simulink model "Validation_Tricopter_Model"  (R2015a)
settings: Solver=ode3  SolverMode=SingleTasking  StartTime=0.0  StopTime=20  FixedStep=T_sim  RelTol=1e-3
PreLoadFcn:
  | LoadLibraries
values from neighbouring files (symbols this model uses):
  a = 10.26    [SetupComplete.m]
  A_x = 0.015    [SetupComplete.m]
  A_y = A_x    (= 0.015)    [SetupComplete.m]
  A_z = 0.16    [SetupComplete.m]
  C_d0 = 0.001193    [SetupComplete.m]
  C_x = 1.2    [SetupComplete.m]
  C_y = C_x    (= 1.2)    [SetupComplete.m]
  C_z = 2.2    [SetupComplete.m]
  CG_0 = [0,0,0.02]'    [SetupComplete.m]
  g = 9.81    [SetupComplete.m]
  h = 0.08    [SetupComplete.m]
  h_FA = 0.02    [SetupComplete.m]
  h_M = 0.064    [SetupComplete.m]
  I_BAC_0 = [ Ix,0,Ixz;0,Iy,0;Ixz,0,Iz]    [SetupComplete.m]
  I_prop = 1/4*M_eq*R^2*diag([1,1,2])    [SetupComplete.m]
  I_tube = [1/2*M_tube*R_tube_eq^2,0,  0  ;           0 ,1/3*M_tube*l_arm^2,0;             0  ,0,1/3*M_tube*l_arm^2]    [SetupComplete.m]
  Initial_Omegas = [1;1;1]*Omega_hover    [Run3Copter.m]
  J_FA = I_prop(1,1) + m_prop*h^2  + m_FA*h_FA^2 + m_M*h_M^2    [SetupComplete.m]
  J_T = J_m+1/2*M_eq*R^2    (= 2.000642e-05)    [SetupComplete.m]
  Ki = lqi(LM_4DOF_aug, Q,R)    [robust_controller.m]
  l = 0.3450    (= 0.345)    [NDI_components.m]    (also in SetupComplete.m; robust_controller.m)
  l_arm = 0.264    [SetupComplete.m]
  m = 3.51    [SetupComplete.m]
  m_0 = 2.61    [SetupComplete.m]
  m_FA = 0.02    [SetupComplete.m]
  m_M = 0.300    (= 0.3)    [SetupComplete.m]
  m_prop = 0.02    [SetupComplete.m]
  R = 0.1778    [SetupComplete.m]    (also in robust_controller.m = eye(4))
  rho = 1.15    [SetupComplete.m]
  sigma = b*c/(pi*R)    (= 0.107416159567)    [SetupComplete.m]
  T_sim = 0.01    [Run3Copter.m]
  theta_0 = 0.38397    [SetupComplete.m]
  theta_1 = -0.2967    [SetupComplete.m]
  trim_simplemodel = [0.589627915568 -2.20656039197 0 0.588313336084 0 0 0.588313330414 0 0]    [trimvalues.mat]
  V_4DOF_last = [0.0122475086001 0.00870447045314 -0.0292257707267 -0.0198753669721 -0.00290766514824 -0.0269511839788 0.0344308792695 -0.0305235710433 -0.0274078219028 -0.0329291952852 -0.0272335702183 -0.00643013158961 ... (1500 elements, 50x30)]    [NN_c_weights.mat]
  v_i0 = sqrt( 1/3*m*g/(2*rho*pi*R^2)  )    [SetupComplete.m]
  W_4DOF_last = [0.0132359246225 -0.0402459595001 -0.0221501781133 0.0046881519205 0.0457506835434 0.0464888535199 -0.0342386918322 0.0470592781761 0.0457166948243 -0.00146243512772 0.0300280468889 -0.0358113661373 ... (204 elements, 4x51)]    [NN_c_weights.mat]
undefined symbols (not defined in the file or in its folder): DOWN_0, EAST_0, Motor, NORTH_0, P_0, Prop, Q_0, R_0, sigmatest, U_0, V_0, v_i_adim, Vx_adim, Vz_adim, W_0
undefined symbols (not defined in the file): Initial_Torques, Rotation_sign, Tau_motors
libraries: simulink x66, XXCopter x32, vrlib x26, simulink_extras x6, Adaptive_FaultTolerantControl x6, qcatlib x4, dspinverses x4, lib_controller x4, aerolib6dofsys x3, aerolibtransform2 x3, aerolib6dof2 x1
(part 7 of 11)

== system Validation_Tricopter_Model/Controller/NDI+CA Controller/4DOF NDI+CA Controller - No massic update/1st order reference model6 ==
  y_ref : Inport
  y_meas : Inport  Port=2
  Bandwidth gain : Gain  Gain=Kb
  Bandwidth gain 1 : Gain  Gain=Kb
  Command FF gain : Gain  Gain=fc
  Command_dot FF gain : Gain  Gain=Kf
  Integral gain : Gain  Gain=fi
  Integrator : Integrator
  Integrator1 : Integrator
  Kref gain : Gain  Gain=Kref
  Sum15 : Sum  Inputs=|+-
  Sum16 : Sum  Inputs=++-
  Sum17 : Sum  Inputs=++|
  Sum5 : Sum  Inputs=|+-
  y_des_dot : Outport
  wires:
  Integral gain/1 -> Integrator1/1
  Bandwidth gain 1/1 -> Integral gain/1
  y_ref/1 -> Sum5/1
  Command_dot FF gain/1 -> Sum17/1
  Command FF gain/1 -> Sum16/1
  Integrator/1 -> Command FF gain/1, Sum15/1, Sum5/2  "y_c"
  y_meas/1 -> Sum16/3, Sum15/2
  Sum16/1 -> Bandwidth gain/1
  Kref gain/1 -> Integrator/1, Command_dot FF gain/1  "y_dot_c"
  Integrator1/1 -> Sum16/2
  Sum17/1 -> y_des_dot/1
  Bandwidth gain/1 -> Sum17/2
  Sum15/1 -> Bandwidth gain 1/1
  Sum5/1 -> Kref gain/1

== system Validation_Tricopter_Model/Controller/NDI+CA Controller/4DOF NDI+CA Controller - No massic update/1st order reference model7 ==
  y_ref : Inport
  y_meas : Inport  Port=2
  Bandwidth gain : Gain  Gain=Kb
  Bandwidth gain 1 : Gain  Gain=Kb
  Command FF gain : Gain  Gain=fc
  Command_dot FF gain : Gain  Gain=Kf
  Integral gain : Gain  Gain=fi
  Integrator : Integrator
  Integrator1 : Integrator
  Kref gain : Gain  Gain=Kref
  Sum15 : Sum  Inputs=|+-
  Sum16 : Sum  Inputs=++-
  Sum17 : Sum  Inputs=++|
  Sum5 : Sum  Inputs=|+-
  y_des_dot : Outport
  wires:
  Sum5/1 -> Kref gain/1
  Sum15/1 -> Bandwidth gain 1/1
  Bandwidth gain/1 -> Sum17/2
  Sum17/1 -> y_des_dot/1
  Integrator1/1 -> Sum16/2
  Kref gain/1 -> Command_dot FF gain/1, Integrator/1  "y_dot_c"
  Sum16/1 -> Bandwidth gain/1
  y_meas/1 -> Sum15/2, Sum16/3
  Integrator/1 -> Sum5/2, Sum15/1, Command FF gain/1  "y_c"
  Command FF gain/1 -> Sum16/1
  Command_dot FF gain/1 -> Sum17/1
  y_ref/1 -> Sum5/1
  Bandwidth gain 1/1 -> Integral gain/1
  Integral gain/1 -> Integrator1/1

== system Validation_Tricopter_Model/Controller/NDI+CA Controller/4DOF NDI+CA Controller - No massic update/Control Allocation 4DOF ==
  Pseudocontrol input : Inport
  Effectiveness control matrix : Inport  Port=2
  Control Allocation 4DOF : Subsystem  VariantControl=(default)
  Pseudoinverse : Subsystem  VariantControl=Variant1
  Control output : Outport

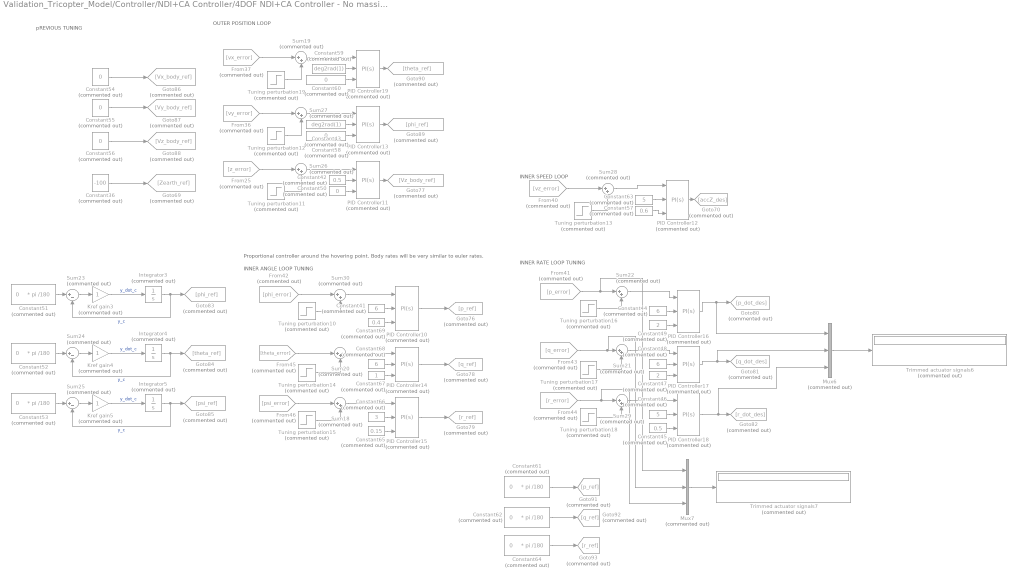
== system Validation_Tricopter_Model/Controller/NDI+CA Controller/4DOF NDI+CA Controller - No massic update/Ideal 4DOF controller ==
  note: OUTER POSITION LOOP
  note: Proportional controller around the hovering point. Body rates will be very similar to euler rates.
  note: INNER RATE LOOP TUNING
  note: INNER ANGLE LOOP TUNING
  note: INNER SPEED LOOP
  note: pREVIOUS TUNING
  Constant36 : Constant  Commented=on  Value=-100
  Constant{41,44,48,68} (4 alike) : Constant  Commented=on  Value=6
  Constant42 : Constant  Commented=on  Value=0.5
  Constant43 : Constant  Commented=on  Value=deg2rad(1)
  Constant45 : Constant  Commented=on  Value=0.5
  Constant46 : Constant  Commented=on  Value=5
  Constant47 : Constant  Commented=on  Value=2
  Constant49 : Constant  Commented=on  Value=2
  Constant{50,54..56,58,60} (6 alike) : Constant  Commented=on  Value=0
  Constant{51..53,61..62,64} (6 alike) : Constant  Commented=on  Value="0     * pi /180"
  Constant57 : Constant  Commented=on  Value=0.6
  Constant59 : Constant  Commented=on  Value=deg2rad(1)
  Constant63 : Constant  Commented=on  Value=5
  Constant65 : Constant  Commented=on  Value=0.15
  Constant66 : Constant  Commented=on  Value=3
  Constant67 : Constant  Commented=on
  Constant69 : Constant  Commented=on  Value=0.4
  From25 : From  Commented=on  GotoTag=z_error
  From36 : From  Commented=on  GotoTag=vy_error
  From37 : From  Commented=on  GotoTag=vx_error
  From40 : From  Commented=on  GotoTag=vz_error
  From41 : From  Commented=on  GotoTag=p_error
  From42 : From  Commented=on  GotoTag=phi_error
  From43 : From  Commented=on  GotoTag=q_error
  From44 : From  Commented=on  GotoTag=r_error
  From45 : From  Commented=on  GotoTag=theta_error
  From46 : From  Commented=on  GotoTag=psi_error
  Goto69 : Goto  Commented=on  GotoTag=Zearth_ref
  Goto70 : Goto  Commented=on  GotoTag=accZ_des
  Goto76 : Goto  Commented=on  GotoTag=p_ref
  Goto77 : Goto  Commented=on  GotoTag=Vz_body_ref
  Goto78 : Goto  Commented=on  GotoTag=q_ref
  Goto79 : Goto  Commented=on  GotoTag=r_ref
  Goto80 : Goto  Commented=on  GotoTag=p_dot_des
  Goto81 : Goto  Commented=on  GotoTag=q_dot_des
  Goto82 : Goto  Commented=on  GotoTag=r_dot_des
  Goto83 : Goto  Commented=on  GotoTag=phi_ref
  Goto84 : Goto  Commented=on  GotoTag=theta_ref
  Goto85 : Goto  Commented=on  GotoTag=psi_ref
  Goto86 : Goto  Commented=on  GotoTag=Vx_body_ref
  Goto87 : Goto  Commented=on  GotoTag=Vy_body_ref
  Goto88 : Goto  Commented=on  GotoTag=Vz_body_ref
  Goto89 : Goto  Commented=on  GotoTag=phi_ref
  Goto90 : Goto  Commented=on  GotoTag=theta_ref
  Goto91 : Goto  Commented=on  GotoTag=p_ref
  Goto92 : Goto  Commented=on  GotoTag=q_ref
  Goto93 : Goto  Commented=on  GotoTag=r_ref
  Integrator3 : Integrator  Commented=on
  Integrator4 : Integrator  Commented=on
  Integrator5 : Integrator  Commented=on
  Kref gain3 : Gain  Commented=on
  Kref gain4 : Gain  Commented=on
  Kref gain5 : Gain  Commented=on
  Mux6 : Mux  Commented=on  Inputs=3
  Mux7 : Mux  Commented=on  Inputs=3
  PID Controller{10..15,18..19} (8 alike) : simulink/Continuous/PID Controller  Commented=on  Controller=PI  TimeDomain=Continuous-time  SampleTime=-1  IntegratorMethod=Forward Euler  FilterMethod=Forward Euler  Form=Parallel  UseFilter=on  ControllerParametersSource=external  P=1  I=1  D=0  N=100  InitialConditionSource=internal  InitialConditionForIntegrator=0  InitialConditionForFilter=0  ExternalReset=none  LimitOutput=off  UpperSaturationLimit=inf  LowerSaturationLimit=-inf  LinearizeAsGain=on  AntiWindupMode=none  Kb=1  TrackingMode=off  Kt=1  PParamMin=[]  PParamMax=[]  IParamMin=[]  IParamMax=[]  DParamMin=[]  DParamMax=[]  NParamMin=[]  NParamMax=[]  KbParamMin=[]  KbParamMax=[]  KtParamMin=[]  KtParamMax=[]  POutMin=[]  POutMax=[]  IOutMin=[]  IOutMax=[]  DOutMin=[]  DOutMax=[]  NOutMin=[]  NOutMax=[]  KbOutMin=[]  KbOutMax=[]  KtOutMin=[]  KtOutMax=[]  IntegratorOutMin=[]  IntegratorOutMax=[]  FilterOutMin=[]  FilterOutMax=[]  SumOutMin=[]  SumOutMax=[]  SumI1OutMin=[]  SumI1OutMax=[]  SumI2OutMin=[]  SumI2OutMax=[]  SumI3OutMin=[]  SumI3OutMax=[]  SumDOutMin=[]  SumDOutMax=[]  SaturationOutMin=[]  SaturationOutMax=[]  IntegratorContinuousStateAttributes=''  IntegratorStateMustResolveToSignalObject=off  IntegratorRTWStateStorageClass=Auto  FilterContinuousStateAttributes=''  FilterStateMustResolveToSignalObject=off  FilterRTWStateStorageClass=Auto  DifferentiatorICPrevScaledInput=0  DifferentiatorOutMin=[]  DifferentiatorOutMax=[]
  PID Controller16 : simulink/Continuous/PID Controller  Commented=on  Controller=PI  TimeDomain=Continuous-time  SampleTime=-1  IntegratorMethod=Forward Euler  FilterMethod=Forward Euler  Form=Parallel  UseFilter=on  ControllerParametersSource=external  P=121.80671459326  I=327.532586687046  D=0  N=100  InitialConditionSource=internal  InitialConditionForIntegrator=0  InitialConditionForFilter=0  ExternalReset=none  LimitOutput=off  UpperSaturationLimit=inf  LowerSaturationLimit=-inf  LinearizeAsGain=on  AntiWindupMode=none  Kb=1  TrackingMode=off  Kt=1  PParamMin=[]  PParamMax=[]  IParamMin=[]  IParamMax=[]  DParamMin=[]  DParamMax=[]  NParamMin=[]  NParamMax=[]  KbParamMin=[]  KbParamMax=[]  KtParamMin=[]  KtParamMax=[]  POutMin=[]  POutMax=[]  IOutMin=[]  IOutMax=[]  DOutMin=[]  DOutMax=[]  NOutMin=[]  NOutMax=[]  KbOutMin=[]  KbOutMax=[]  KtOutMin=[]  KtOutMax=[]  IntegratorOutMin=[]  IntegratorOutMax=[]  FilterOutMin=[]  FilterOutMax=[]  SumOutMin=[]  SumOutMax=[]  SumI1OutMin=[]  SumI1OutMax=[]  SumI2OutMin=[]  SumI2OutMax=[]  SumI3OutMin=[]  SumI3OutMax=[]  SumDOutMin=[]  SumDOutMax=[]  SaturationOutMin=[]  SaturationOutMax=[]  IntegratorContinuousStateAttributes=''  IntegratorStateMustResolveToSignalObject=off  IntegratorRTWStateStorageClass=Auto  FilterContinuousStateAttributes=''  FilterStateMustResolveToSignalObject=off  FilterRTWStateStorageClass=Auto  DifferentiatorICPrevScaledInput=0  DifferentiatorOutMin=[]  DifferentiatorOutMax=[]
  PID Controller17 : simulink/Continuous/PID Controller  Commented=on  Controller=PI  TimeDomain=Continuous-time  SampleTime=-1  IntegratorMethod=Forward Euler  FilterMethod=Forward Euler  Form=Parallel  UseFilter=on  ControllerParametersSource=external  P=244.169484479421  I=1759.80724182952  D=0  N=100  InitialConditionSource=internal  InitialConditionForIntegrator=0  InitialConditionForFilter=0  ExternalReset=none  LimitOutput=off  UpperSaturationLimit=inf  LowerSaturationLimit=-inf  LinearizeAsGain=on  AntiWindupMode=none  Kb=1  TrackingMode=off  Kt=1  PParamMin=[]  PParamMax=[]  IParamMin=[]  IParamMax=[]  DParamMin=[]  DParamMax=[]  NParamMin=[]  NParamMax=[]  KbParamMin=[]  KbParamMax=[]  KtParamMin=[]  KtParamMax=[]  POutMin=[]  POutMax=[]  IOutMin=[]  IOutMax=[]  DOutMin=[]  DOutMax=[]  NOutMin=[]  NOutMax=[]  KbOutMin=[]  KbOutMax=[]  KtOutMin=[]  KtOutMax=[]  IntegratorOutMin=[]  IntegratorOutMax=[]  FilterOutMin=[]  FilterOutMax=[]  SumOutMin=[]  SumOutMax=[]  SumI1OutMin=[]  SumI1OutMax=[]  SumI2OutMin=[]  SumI2OutMax=[]  SumI3OutMin=[]  SumI3OutMax=[]  SumDOutMin=[]  SumDOutMax=[]  SaturationOutMin=[]  SaturationOutMax=[]  IntegratorContinuousStateAttributes=''  IntegratorStateMustResolveToSignalObject=off  IntegratorRTWStateStorageClass=Auto  FilterContinuousStateAttributes=''  FilterStateMustResolveToSignalObject=off  FilterRTWStateStorageClass=Auto  DifferentiatorICPrevScaledInput=0  DifferentiatorOutMin=[]  DifferentiatorOutMax=[]
  Sum{18..22,26..30} (10 alike) : Sum  Commented=on  Inputs=|++
  Sum23 : Sum  Commented=on  Inputs=|+-
  Sum24 : Sum  Commented=on  Inputs=|+-
  Sum25 : Sum  Commented=on  Inputs=|+-
  Trimmed actuator signals6 : Display  Commented=on
  Trimmed actuator signals7 : Display  Commented=on
  Tuning perturbation{10,15..16,18} (4 alike) : Step  Commented=on  Time=20  After=3*pi/180  SampleTime=0
  Tuning perturbation{11..13,19} (4 alike) : Step  Commented=on  Time=20  SampleTime=0
  Tuning perturbation14 : Step  Commented=on  Time=20  After=-3*pi/180  SampleTime=0
  Tuning perturbation17 : Step  Commented=on  Time=20  After=-3*pi/180  SampleTime=0
  wires:
  From42/1 -> Sum30/1
  Constant56/1 -> Goto88/1
  Constant55/1 -> Goto87/1
  Constant54/1 -> Goto86/1
  PID Controller12/1 -> Goto70/1
  Mux6/1 -> Trimmed actuator signals6/1
  Tuning perturbation17/1 -> Sum21/2
  Constant59/1 -> PID Controller19/2
  PID Controller13/1 -> Goto89/1
  Tuning perturbation12/1 -> Sum27/2
  From36/1 -> Sum27/1
  Sum27/1 -> PID Controller13/1
  Constant58/1 -> PID Controller13/3
  PID Controller16/1 -> Goto80/1, Mux6/1
  Tuning perturbation14/1 -> Sum20/2
  Tuning perturbation10/1 -> Sum30/2
  Tuning perturbation15/1 -> Sum18/2
  Sum20/1 -> PID Controller14/1
  Constant66/1 -> PID Controller15/2
  PID Controller15/1 -> Goto79/1
  PID Controller14/1 -> Goto78/1
  PID Controller10/1 -> Goto76/1
  Tuning perturbation13/1 -> Sum28/2
  From40/1 -> Sum28/1
  Constant52/1 -> Sum24/1
  Constant61/1 -> Goto91/1
  Constant45/1 -> PID Controller18/3
  Constant49/1 -> PID Controller16/3
  Sum25/1 -> Kref gain5/1
  Kref gain5/1 -> Integrator5/1  "y_dot_c"
  From43/1 -> Sum21/1, Mux7/2
  From41/1 -> Sum22/1, Mux7/1
  From46/1 -> Sum18/1
  From45/1 -> Sum20/1
  Sum28/1 -> PID Controller12/1
  Constant57/1 -> PID Controller12/3
  Constant63/1 -> PID Controller12/2
  Constant64/1 -> Goto93/1
  Constant62/1 -> Goto92/1
  Constant42/1 -> PID Controller11/2
  Constant36/1 -> Goto69/1
  Constant44/1 -> PID Controller16/2
  Mux7/1 -> Trimmed actuator signals7/1
  From44/1 -> Sum29/1, Mux7/3
  Constant48/1 -> PID Controller17/2
  Constant46/1 -> PID Controller18/2
  PID Controller18/1 -> Goto82/1, Mux6/3
  PID Controller17/1 -> Goto81/1, Mux6/2
  Integrator3/1 -> Goto83/1, Sum23/2  "y_c"
  Constant51/1 -> Sum23/1
  PID Controller19/1 -> Goto90/1
  Tuning perturbation19/1 -> Sum19/2
  From37/1 -> Sum19/1
  Sum19/1 -> PID Controller19/1
  Constant60/1 -> PID Controller19/3
  Constant43/1 -> PID Controller13/2
  PID Controller11/1 -> Goto77/1
  Tuning perturbation11/1 -> Sum26/2
  From25/1 -> Sum26/1
  Sum26/1 -> PID Controller11/1
  Constant50/1 -> PID Controller11/3
  Integrator5/1 -> Goto85/1, Sum25/2  "y_c"
  Constant53/1 -> Sum25/1
  Sum24/1 -> Kref gain4/1
  Kref gain4/1 -> Integrator4/1  "y_dot_c"
  Sum23/1 -> Kref gain3/1
  Kref gain3/1 -> Integrator3/1  "y_dot_c"
  Tuning perturbation16/1 -> Sum22/2
  Tuning perturbation18/1 -> Sum29/2
  Sum21/1 -> PID Controller17/1
  Sum29/1 -> PID Controller18/1
  Sum22/1 -> PID Controller16/1
  Constant47/1 -> PID Controller17/3
  Sum18/1 -> PID Controller15/1
  Sum30/1 -> PID Controller10/1
  Constant67/1 -> PID Controller14/3
  Constant69/1 -> PID Controller10/3
  Constant41/1 -> PID Controller10/2
  Constant68/1 -> PID Controller14/2
  Constant65/1 -> PID Controller15/3
  Integrator4/1 -> Sum24/2, Goto84/1  "y_c"

== system Validation_Tricopter_Model/3 Copter Complete/Arms Dynamics: Forces and Moments/4 DOF Arms Dynamics: Forces and Moments1/4 DOF Arms Dynamics: Forces and Moments1/Arm Dynamics ==
  note: Motor-Propeller Coupling: Propeller Torque
  Throttle [0-1] : Inport
  Comm Angles (rad) : Inport  Port=2
  Omega_Initial : Inport  Port=3
  h_ground : Inport  Port=4
  omega_b : Inport  Port=5
  V_b : Inport  Port=6
  Aerodynamics Propeller : Subsystem  TreatAsAtomicUnit=on  mask{Rot_sign=Rot_sign}
      mask prompts: Rot_sign "Rotation Sign"
      settings: MinAlgLoopOccurrences=on
      mask TypeOptions Rot_sign: Rotation_sign/Value
  Arms Kinematics : Subsystem  AncestorBlock=XXCopter/Arms Kinematics  TreatAsAtomicUnit=on  mask{Arm_number=arm_num, Arm_hub_position=arm_hub_pos, eta_dir=eta_dir, gamma_dir=gamma_dir, h_prop=h}
      mask prompts: Arm_number "Arm number (1,2 or 3)"; Arm_hub_position "Arm Hub position"; eta_dir "eta direcction"; gamma_dir "gamma diretion"; h_prop "h of propeller hub"
      mask help:
      | If Arm number 1 (Forward one)
      | eta_dir=[1,0,0]
      | gamma_dir=[0,1,0]
      |
      | If Arm number 2 or 3 (rear ones)
      | eta_dir=[0,1,0]
      | gamma_dir=[1,0,0]
      mask TypeOptions Arm_number: Arm_no/Value
      mask TypeOptions Arm_hub_position: Hub_position/Value
      mask TypeOptions eta_dir: eta_dir/Gain
      mask TypeOptions gamma_dir: gamma_dir/Gain
      mask TypeOptions h_prop: h arm/Value
  Cross Product : vrlib/Utilities/Cross Product
  Display : Display
  ESC+Motor Dynamcis : XXCopter/ESC+Motor Dynamcis  Inertia_swithc_var=Motor+Prop  J_T=J_T  tau=tau
  Ground : Ground
  Gyroscopic Moments : Subsystem  AncestorBlock=XXCopter/Gyroscopic Moments  TreatAsAtomicUnit=on  mask{Arm_axis=[l_arm;0;0], Rot_sign=Rot_sign, eta_dir=eta_dir, gamma_dir=gamma_dir, J_T=J_T, J_FA=J_FA}
      mask prompts: Arm_axis "Arm axis from Servo origin"; Rot_sign "Rotation sign"; eta_dir "eta direction"; gamma_dir "gamma direction"; J_T "Inertia Motor+Prop"; J_FA "Inertia Foreamr"
      mask TypeOptions Arm_axis: Hub_position/Value
      mask TypeOptions Rot_sign: Rotation_sign/Value | Rotation_sign1/Value
      mask TypeOptions eta_dir: eta_dir/Gain | eta_dir1/Gain
      mask TypeOptions gamma_dir: gamma_dir/Gain | gamma_dir1/Gain
      mask TypeOptions J_T: Propeller and motor inertia/Value | Propeller and motor inertia1/Value
      mask TypeOptions J_FA: Forearm Inertia/Value | Forearm Inertia1/Value
  Initial_torque : Memory  X0=Torq_ini
  Math Function : Math  Operator=square  SaturateOnIntegerOverflow=on
  Math Function1 : Math  Operator=sqrt  SaturateOnIntegerOverflow=on
  Math Function2 : Math  Operator=square  SaturateOnIntegerOverflow=on
  Math Function3 : Math  Operator=sqrt  SaturateOnIntegerOverflow=on
  Mux : Mux  Inputs=2
  Scope : Scope
      settings: YMin=-25  SaveName=ScopeData10
  Servos Dynamics : Subsystem  AncestorBlock=XXCopter/Servos Dynamics  TreatAsAtomicUnit=on  mask{omega_n=omega_n, xi=xi, derv_param=c, init_eta=init_eta, init_gamma=0}
      mask prompts: omega_n "Servo natural freq (rad/s) omega_n"; xi "Servo damping xi"; derv_param "Derivative parameter"; init_eta "Initial eta (rad)"; init_gamma "Initial gamma (rad)"
      mask TypeOptions init_eta: init_eta/Value | init_eta1/Value
      mask TypeOptions init_gamma: init_gamma/Value | init_gamma1/Value
  Sum of Elements : Sum  Inputs=+
  Sum of Elements1 : Sum  Inputs=+
  Total moments : Sum
  V^A (m/s) : Sum  Inputs=+++
  initial_omega : Memory  X0=Omega_ini
  omega_A : Sum
  omega_b1 : InportShadow  Port=5
  Forces : Outport
  Moments : Outport  Port=2
  Omega_out : Outport  Port=3
  Omega_dot_out : Outport  Port=4
  T_FaFb : Outport  Port=5
  Angles (rad) : Outport  Port=6
  r_p : Outport  Port=7
  wires:
  initial_omega/1 -> ESC+Motor Dynamcis/2
  Initial_torque/1 -> ESC+Motor Dynamcis/4
  Aerodynamics Propeller/1(Prop_Torque_out) -> Initial_torque/1
  Total moments/1 -> Moments/1
  Gyroscopic Moments/1(M_gyro @Fb) -> Math Function2/1, Total moments/2
  Aerodynamics Propeller/3(Moments_prop @Fb) -> Math Function/1, Total moments/1
  Ground/1 -> Servos Dynamics/2(Torques?)
  Servos Dynamics/3(Angles_dot_dot (rad/s^2)) -> Gyroscopic Moments/5(Angles_dot _dot(rad/s^2))
  omega_A/1 -> Gyroscopic Moments/2(omega_A  (rad/s))
  omega_b1/1 -> omega_A/2, Gyroscopic Moments/3(omega_b  (rad/s))
  Arms Kinematics/4(omega_Ab (rad/s)) -> omega_A/1
  Servos Dynamics/2(Angles_dot (rad/s)) -> Arms Kinematics/2(Angles_dot (rad/s)), Gyroscopic Moments/4(Angles_dot (rad/s))
  Aerodynamics Propeller/2(Forces_prop @Fb) -> Scope/1, Forces/1
  Arms Kinematics/1(r_p (m)) -> r_p/1, Cross Product/2, Aerodynamics Propeller/3(r_p)
  Arms Kinematics/3(T_F_a,Fb) -> T_FaFb/1, Aerodynamics Propeller/5(T_FaFb), Gyroscopic Moments/1(T_FAFb)
  V^A (m/s)/1 -> Aerodynamics Propeller/4(V^A)
  Arms Kinematics/2(r_p_dot (m/s)) -> V^A (m/s)/3
  V_b/1 -> V^A (m/s)/1
  Cross Product/1 -> V^A (m/s)/2
  omega_b/1 -> Cross Product/1
  Servos Dynamics/1(Angles Arms (rad)) -> Angles (rad)/1, Arms Kinematics/1(Angles (rad))
  Comm Angles (rad)/1 -> Servos Dynamics/1(Com Angles (rad))
  h_ground/1 -> Aerodynamics Propeller/2(h_ground)
  ESC+Motor Dynamcis/1 -> Aerodynamics Propeller/1(Omega), Omega_out/1, Gyroscopic Moments/6(Omega (rad/s)), initial_omega/1  "Omega"
  ESC+Motor Dynamcis/2 -> Omega_dot_out/1, Gyroscopic Moments/7(Omega_dot (rad/s^2))  "Omega_dot"
  Omega_Initial/1 -> ESC+Motor Dynamcis/3
  Throttle [0-1]/1 -> ESC+Motor Dynamcis/1
  Mux/1 -> Display/1
  Sum of Elements/1 -> Math Function1/1
  Math Function/1 -> Sum of Elements/1
  Math Function1/1 -> Mux/1
  Sum of Elements1/1 -> Math Function3/1
  Math Function2/1 -> Sum of Elements1/1
  Math Function3/1 -> Mux/2

== system Validation_Tricopter_Model/3 Copter Complete/Arms Dynamics: Forces and Moments/4 DOF Arms Dynamics: Forces and Moments1/4 DOF Arms Dynamics: Forces and Moments1/Arm Dynamics1 ==
  note: Motor-Propeller Coupling: Propeller Torque
  Throttle [0-1] : Inport
  Comm Angles (rad) : Inport  Port=2
  Omega_Initial : Inport  Port=3
  h_ground : Inport  Port=4
  omega_b : Inport  Port=5
  V_b : Inport  Port=6
  Aerodynamics Propeller : Subsystem  TreatAsAtomicUnit=on  mask{Rot_sign=Rot_sign}
      mask prompts: Rot_sign "Rotation Sign"
      settings: MinAlgLoopOccurrences=on
      mask TypeOptions Rot_sign: Rotation_sign/Value
  Arms Kinematics : Subsystem  AncestorBlock=XXCopter/Arms Kinematics  TreatAsAtomicUnit=on  mask{Arm_number=arm_num, Arm_hub_position=arm_hub_pos, eta_dir=eta_dir, gamma_dir=gamma_dir, h_prop=h}
      mask prompts: Arm_number "Arm number (1,2 or 3)"; Arm_hub_position "Arm Hub position"; eta_dir "eta direcction"; gamma_dir "gamma diretion"; h_prop "h of propeller hub"
      mask help:
      | If Arm number 1 (Forward one)
      | eta_dir=[1,0,0]
      | gamma_dir=[0,1,0]
      |
      | If Arm number 2 or 3 (rear ones)
      | eta_dir=[0,1,0]
      | gamma_dir=[1,0,0]
      mask TypeOptions Arm_number: Arm_no/Value
      mask TypeOptions Arm_hub_position: Hub_position/Value
      mask TypeOptions eta_dir: eta_dir/Gain
      mask TypeOptions gamma_dir: gamma_dir/Gain
      mask TypeOptions h_prop: h arm/Value
  Cross Product : vrlib/Utilities/Cross Product
  Display : Display
  ESC+Motor Dynamcis : XXCopter/ESC+Motor Dynamcis  Inertia_swithc_var=Motor+Prop  J_T=J_T  tau=tau
  Ground : Ground
  Gyroscopic Moments : XXCopter/Gyroscopic Moments  arm_axis=arm_axis  Rot_sign=Rot_sign  eta_dir=eta_dir  gamma_dir=gamma_dir  J_T=J_T  J_FA=J_FA
  Initial_torque : Memory  X0=Torq_ini
  Scope : Scope
      settings: YMin=-30  YMax=10  SaveName=ScopeData11
  Scope1 : Scope
      settings: YMin=-1.5  YMax=1  SaveName=ScopeData12
  Servos Dynamics : XXCopter/Servos Dynamics  omega_n=omega_n  xi=xi  derv_param=c  init_eta=init_eta  init_gamma=0
      link override eta_1: Numerator=0  Denominator=1
      link override eta_2: Numerator=0  Denominator=1
  Total moments : Sum
  V^A (m/s) : Sum  Inputs=+++
  initial_omega : Memory  X0=Omega_ini
  omega_A : Sum
  omega_b1 : InportShadow  Port=5
  Forces : Outport
  Moments : Outport  Port=2
  Omega_out : Outport  Port=3
  Omega_dot_out : Outport  Port=4
  T_FaFb : Outport  Port=5
  Angles (rad) : Outport  Port=6
  r_p : Outport  Port=7
  wires:
  initial_omega/1 -> ESC+Motor Dynamcis/2
  Initial_torque/1 -> ESC+Motor Dynamcis/4
  Aerodynamics Propeller/1(Prop_Torque_out) -> Initial_torque/1
  Total moments/1 -> Moments/1
  Gyroscopic Moments/1 -> Total moments/2
  Aerodynamics Propeller/3(Moments_prop @Fb) -> Total moments/1
  Ground/1 -> Servos Dynamics/2
  Servos Dynamics/3 -> Gyroscopic Moments/5
  omega_A/1 -> Gyroscopic Moments/2
  omega_b1/1 -> omega_A/2, Gyroscopic Moments/3
  Arms Kinematics/4(omega_Ab (rad/s)) -> omega_A/1
  Servos Dynamics/2 -> Arms Kinematics/2(Angles_dot (rad/s)), Gyroscopic Moments/4
  Aerodynamics Propeller/2(Forces_prop @Fb) -> Scope/1, Forces/1
  Arms Kinematics/1(r_p (m)) -> r_p/1, Cross Product/2, Aerodynamics Propeller/3(r_p)
  Arms Kinematics/3(T_F_a,Fb) -> T_FaFb/1, Aerodynamics Propeller/5(T_FaFb), Display/1, Gyroscopic Moments/1
  V^A (m/s)/1 -> Scope1/1, Aerodynamics Propeller/4(V^A)
  Arms Kinematics/2(r_p_dot (m/s)) -> V^A (m/s)/3
  V_b/1 -> V^A (m/s)/1
  Cross Product/1 -> V^A (m/s)/2
  omega_b/1 -> Cross Product/1
  Servos Dynamics/1 -> Angles (rad)/1, Arms Kinematics/1(Angles (rad))
  Comm Angles (rad)/1 -> Servos Dynamics/1
  h_ground/1 -> Aerodynamics Propeller/2(h_ground)
  ESC+Motor Dynamcis/1 -> Aerodynamics Propeller/1(Omega), Omega_out/1, Gyroscopic Moments/6, initial_omega/1  "Omega"
  ESC+Motor Dynamcis/2 -> Omega_dot_out/1, Gyroscopic Moments/7  "Omega_dot"
  Omega_Initial/1 -> ESC+Motor Dynamcis/3
  Throttle [0-1]/1 -> ESC+Motor Dynamcis/1

== system Validation_Tricopter_Model/3 Copter Complete/Arms Dynamics: Forces and Moments/4 DOF Arms Dynamics: Forces and Moments1/4 DOF Arms Dynamics: Forces and Moments1/Arm Dynamics2 ==
  note: Motor-Propeller Coupling: Propeller Torque
  Throttle [0-1] : Inport
  Comm Angles (rad) : Inport  Port=2
  Omega_Initial : Inport  Port=3
  h_ground : Inport  Port=4
  omega_b : Inport  Port=5
  V_b : Inport  Port=6
  Aerodynamics Propeller : Subsystem  TreatAsAtomicUnit=on  mask{Rot_sign=Rot_sign}
      mask prompts: Rot_sign "Rotation Sign"
      settings: MinAlgLoopOccurrences=on
      mask TypeOptions Rot_sign: Rotation_sign/Value
  Arms Kinematics : Subsystem  AncestorBlock=XXCopter/Arms Kinematics  TreatAsAtomicUnit=on  mask{Arm_number=arm_num, Arm_hub_position=arm_hub_pos, eta_dir=eta_dir, gamma_dir=gamma_dir, h_prop=h}
      mask prompts: Arm_number "Arm number (1,2 or 3)"; Arm_hub_position "Arm Hub position"; eta_dir "eta direcction"; gamma_dir "gamma diretion"; h_prop "h of propeller hub"
      mask help:
      | If Arm number 1 (Forward one)
      | eta_dir=[1,0,0]
      | gamma_dir=[0,1,0]
      |
      | If Arm number 2 or 3 (rear ones)
      | eta_dir=[0,1,0]
      | gamma_dir=[1,0,0]
      mask TypeOptions Arm_number: Arm_no/Value
      mask TypeOptions Arm_hub_position: Hub_position/Value
      mask TypeOptions eta_dir: eta_dir/Gain
      mask TypeOptions gamma_dir: gamma_dir/Gain
      mask TypeOptions h_prop: h arm/Value
  Cross Product : vrlib/Utilities/Cross Product
  ESC+Motor Dynamcis : XXCopter/ESC+Motor Dynamcis  Inertia_swithc_var=Motor+Prop  J_T=J_T  tau=tau
  Ground : Ground
  Gyroscopic Moments : XXCopter/Gyroscopic Moments  arm_axis=arm_axis  Rot_sign=Rot_sign  eta_dir=eta_dir  gamma_dir=gamma_dir  J_T=J_T  J_FA=J_FA
  Initial_torque : Memory  X0=Torq_ini
  Servos Dynamics : Subsystem  AncestorBlock=XXCopter/Servos Dynamics  TreatAsAtomicUnit=on  mask{omega_n=omega_n, xi=xi, derv_param=c, init_eta=init_eta, init_gamma=0}
      mask prompts: omega_n "Servo natural freq (rad/s) omega_n"; xi "Servo damping xi"; derv_param "Derivative parameter"; init_eta "Initial eta (rad)"; init_gamma "Initial gamma (rad)"
      mask TypeOptions init_eta: init_eta/Value | init_eta1/Value
      mask TypeOptions init_gamma: init_gamma/Value | init_gamma1/Value
  Total moments : Sum
  V^A (m/s) : Sum  Inputs=+++
  initial_omega : Memory  X0=Omega_ini
  omega_A : Sum
  omega_b1 : InportShadow  Port=5
  Forces : Outport
  Moments : Outport  Port=2
  Omega_out : Outport  Port=3
  Omega_dot_out : Outport  Port=4
  T_FaFb : Outport  Port=5
  Angles (rad) : Outport  Port=6
  r_p : Outport  Port=7
  wires:
  initial_omega/1 -> ESC+Motor Dynamcis/2
  Initial_torque/1 -> ESC+Motor Dynamcis/4
  Aerodynamics Propeller/1(Prop_Torque_out) -> Initial_torque/1
  Total moments/1 -> Moments/1
  Gyroscopic Moments/1 -> Total moments/2
  Aerodynamics Propeller/3(Moments_prop @Fb) -> Total moments/1
  Ground/1 -> Servos Dynamics/2(Torques?)
  Servos Dynamics/3(Angles_dot_dot (rad/s^2)) -> Gyroscopic Moments/5
  omega_A/1 -> Gyroscopic Moments/2
  omega_b1/1 -> omega_A/2, Gyroscopic Moments/3
  Arms Kinematics/4(omega_Ab (rad/s)) -> omega_A/1
  Servos Dynamics/2(Angles_dot (rad/s)) -> Arms Kinematics/2(Angles_dot (rad/s)), Gyroscopic Moments/4
  Aerodynamics Propeller/2(Forces_prop @Fb) -> Forces/1
  Arms Kinematics/1(r_p (m)) -> r_p/1, Cross Product/2, Aerodynamics Propeller/3(r_p)
  Arms Kinematics/3(T_F_a,Fb) -> T_FaFb/1, Aerodynamics Propeller/5(T_FaFb), Gyroscopic Moments/1
  V^A (m/s)/1 -> Aerodynamics Propeller/4(V^A)
  Arms Kinematics/2(r_p_dot (m/s)) -> V^A (m/s)/3
  V_b/1 -> V^A (m/s)/1
  Cross Product/1 -> V^A (m/s)/2
  omega_b/1 -> Cross Product/1
  Servos Dynamics/1(Angles Arms (rad)) -> Angles (rad)/1, Arms Kinematics/1(Angles (rad))
  Comm Angles (rad)/1 -> Servos Dynamics/1(Com Angles (rad))
  h_ground/1 -> Aerodynamics Propeller/2(h_ground)
  ESC+Motor Dynamcis/1 -> Aerodynamics Propeller/1(Omega), Omega_out/1, Gyroscopic Moments/6, initial_omega/1  "Omega"
  ESC+Motor Dynamcis/2 -> Omega_dot_out/1, Gyroscopic Moments/7  "Omega_dot"
  Omega_Initial/1 -> ESC+Motor Dynamcis/3
  Throttle [0-1]/1 -> ESC+Motor Dynamcis/1

== system Validation_Tricopter_Model/3 Copter Complete/Arms Dynamics: Forces and Moments/9 DOF Arms Dynamics: Forces and Moments/9 DOF Arms Dynamics: Forces and Moments/Arm Dynamics ==
  note: Motor-Propeller Coupling: Propeller Torque
  Throttle [0-1] : Inport
  Comm Angles (rad) : Inport  Port=2
  Omega_Initial : Inport  Port=3
  h_ground : Inport  Port=4
  omega_b : Inport  Port=5
  V_b : Inport  Port=6
  Aerodynamics Propeller : Subsystem  TreatAsAtomicUnit=on  mask{Rot_sign=Rot_sign}
      mask prompts: Rot_sign "Rotation Sign"
      settings: MinAlgLoopOccurrences=on
      mask TypeOptions Rot_sign: Rotation_sign/Value
  Arms Kinematics : Subsystem  AncestorBlock=XXCopter/Arms Kinematics  TreatAsAtomicUnit=on  mask{Arm_number=arm_num, Arm_hub_position=arm_hub_pos, eta_dir=eta_dir, gamma_dir=gamma_dir, h_prop=h}
      mask prompts: Arm_number "Arm number (1,2 or 3)"; Arm_hub_position "Arm Hub position"; eta_dir "eta direcction"; gamma_dir "gamma diretion"; h_prop "h of propeller hub"
      mask help:
      | If Arm number 1 (Forward one)
      | eta_dir=[1,0,0]
      | gamma_dir=[0,1,0]
      |
      | If Arm number 2 or 3 (rear ones)
      | eta_dir=[0,1,0]
      | gamma_dir=[1,0,0]
      mask TypeOptions Arm_number: Arm_no/Value
      mask TypeOptions Arm_hub_position: Hub_position/Value
      mask TypeOptions eta_dir: eta_dir/Gain
      mask TypeOptions gamma_dir: gamma_dir/Gain
      mask TypeOptions h_prop: h arm/Value
  Cross Product : vrlib/Utilities/Cross Product
  ESC+Motor Dynamcis : XXCopter/ESC+Motor Dynamcis  Inertia_swithc_var=None  J_T=J_T  tau=tau
  F_b->F_A : Product  Multiplication=Matrix(*)
  Ground : Ground
  Gyroscopic Moments : Subsystem  AncestorBlock=XXCopter/Gyroscopic Moments  TreatAsAtomicUnit=on  mask{arm_axis=[l_arm;0;0], Rot_sign=Rot_sign, eta_dir=eta_dir, gamma_dir=gamma_dir, J_T=J_T, J_FA=J_FA}
      mask prompts: arm_axis "Arm axis from Servo origin"; Rot_sign "Rotation sign"; eta_dir "eta direction"; gamma_dir "gamma direction"; J_T "Inertia Motor+Prop"; J_FA "Inertia Foreamr"
      mask TypeOptions arm_axis: arm_axis/Value
      mask TypeOptions Rot_sign: Rotation_sign/Value | Rotation_sign1/Value
      mask TypeOptions eta_dir: eta_dir/Gain | eta_dir1/Gain
      mask TypeOptions gamma_dir: gamma_dir/Gain | gamma_dir1/Gain
      mask TypeOptions J_T: Propeller and motor inertia/Value | Propeller and motor inertia1/Value
      mask TypeOptions J_FA: Forearm Inertia/Value | Forearm Inertia1/Value
  Initial_torque : Memory  X0=Torq_ini
  Math Function2 : Math  Operator=square  SaturateOnIntegerOverflow=on
  Math Function3 : Math  Operator=sqrt  SaturateOnIntegerOverflow=on
  Math Function4 : Math  Operator=square  SaturateOnIntegerOverflow=on
  Math Function5 : Math  Operator=sqrt  SaturateOnIntegerOverflow=on
  Mux : Mux  Inputs=2
  Mux2 : Mux  Inputs=2
  Permute Dimensions : PermuteDimensions
  Scope : Scope
      settings: TimeRange=20  YMin=-20  SaveName=TestMotor
  Scope1 : Scope
      settings: YMin=-2  YMax=6.5  SaveName=ScopeData2
  Scope2 : Scope
      settings: YMin=-2  YMax=6.5  SaveName=ScopeData13
  Servos Dynamics : XXCopter/Servos Dynamics  omega_n=omega_n  xi=xi  derv_param=c  init_eta=init_eta  init_gamma=0
  Sum of Elements1 : Sum  Inputs=+
  Sum of Elements2 : Sum  Inputs=+
  To File : ToFile  Filename=gyro_comparison.mat  MatrixName=gyro_comp  SaveFormat=Timeseries
  Total moments : Sum
  V^A (m/s) : Sum  Inputs=+++
  initial_omega : Memory  X0=Omega_ini
  omega_A : Sum
  omega_b1 : InportShadow  Port=5
  Forces : Outport
  Moments : Outport  Port=2
  Omega_out : Outport  Port=3
  Omega_dot_out : Outport  Port=4
  T_FaFb : Outport  Port=5
  Angles (rad) : Outport  Port=6
  r_p : Outport  Port=7
  wires:
  F_b->F_A/1 -> Aerodynamics Propeller/4(V^A)
  Permute Dimensions/1 -> F_b->F_A/1
  V^A (m/s)/1 -> F_b->F_A/2
  initial_omega/1 -> ESC+Motor Dynamcis/2
  Initial_torque/1 -> ESC+Motor Dynamcis/4
  Aerodynamics Propeller/1(Prop_Torque_out) -> Initial_torque/1
  Total moments/1 -> Moments/1
  Gyroscopic Moments/1(M_gyro @Fb) -> Mux/2, Math Function2/1, Total moments/2
  Ground/1 -> Servos Dynamics/2
  Servos Dynamics/3 -> Gyroscopic Moments/5(Angles_dot _dot(rad/s^2))
  omega_A/1 -> Gyroscopic Moments/2(omega_A  (rad/s))
  omega_b1/1 -> omega_A/2, Gyroscopic Moments/3(omega_b  (rad/s))
  Arms Kinematics/4(omega_Ab (rad/s)) -> omega_A/1
  Servos Dynamics/2 -> Arms Kinematics/2(Angles_dot (rad/s)), Gyroscopic Moments/4(Angles_dot (rad/s))
  Aerodynamics Propeller/2(Forces_prop @Fb) -> Scope/1, Forces/1
  Arms Kinematics/1(r_p (m)) -> r_p/1, Cross Product/2, Aerodynamics Propeller/3(r_p)
  Arms Kinematics/2(r_p_dot (m/s)) -> V^A (m/s)/3
  V_b/1 -> V^A (m/s)/1
  Cross Product/1 -> V^A (m/s)/2
  omega_b/1 -> Cross Product/1
  Servos Dynamics/1 -> Angles (rad)/1, Arms Kinematics/1(Angles (rad))
  Comm Angles (rad)/1 -> Servos Dynamics/1
  h_ground/1 -> Aerodynamics Propeller/2(h_ground)
  ESC+Motor Dynamcis/1 -> Aerodynamics Propeller/1(Omega), Omega_out/1, Gyroscopic Moments/6(Omega (rad/s)), initial_omega/1  "Omega"
  ESC+Motor Dynamcis/2 -> Omega_dot_out/1, Gyroscopic Moments/7(Omega_dot (rad/s^2))  "Omega_dot"
  Omega_Initial/1 -> ESC+Motor Dynamcis/3
  Throttle [0-1]/1 -> ESC+Motor Dynamcis/1
  Arms Kinematics/3(T_F_a,Fb) -> Permute Dimensions/1, T_FaFb/1, Aerodynamics Propeller/5(T_FaFb), Gyroscopic Moments/1(T_FAFb)
  Mux/1 -> Scope1/1
  Sum of Elements1/1 -> Math Function3/1
  Math Function2/1 -> Sum of Elements1/1
  Math Function4/1 -> Sum of Elements2/1
  Sum of Elements2/1 -> Math Function5/1
  Math Function5/1 -> Mux2/1  "aero"
  Math Function3/1 -> Mux2/2  "gyro"
  Aerodynamics Propeller/3(Moments_prop @Fb) -> Math Function4/1, Mux/1, Total moments/1
  Mux2/1 -> To File/1, Scope2/1

== system Validation_Tricopter_Model/3 Copter Complete/Arms Dynamics: Forces and Moments/9 DOF Arms Dynamics: Forces and Moments/9 DOF Arms Dynamics: Forces and Moments/Arm Dynamics1 ==
  note: Motor-Propeller Coupling: Propeller Torque
  Throttle [0-1] : Inport
  Comm Angles (rad) : Inport  Port=2
  Omega_Initial : Inport  Port=3
  h_ground : Inport  Port=4
  omega_b : Inport  Port=5
  V_b : Inport  Port=6
  Aerodynamics Propeller : Subsystem  TreatAsAtomicUnit=on  mask{Rot_sign=Rot_sign}
      mask prompts: Rot_sign "Rotation Sign"
      settings: MinAlgLoopOccurrences=on
      mask TypeOptions Rot_sign: Rotation_sign/Value
  Arms Kinematics : Subsystem  AncestorBlock=XXCopter/Arms Kinematics  TreatAsAtomicUnit=on  mask{Arm_number=arm_num, Arm_hub_position=arm_hub_pos, eta_dir=eta_dir, gamma_dir=gamma_dir, h_prop=h}
      mask prompts: Arm_number "Arm number (1,2 or 3)"; Arm_hub_position "Arm Hub position"; eta_dir "eta direcction"; gamma_dir "gamma diretion"; h_prop "h of propeller hub"
      mask help:
      | If Arm number 1 (Forward one)
      | eta_dir=[1,0,0]
      | gamma_dir=[0,1,0]
      |
      | If Arm number 2 or 3 (rear ones)
      | eta_dir=[0,1,0]
      | gamma_dir=[1,0,0]
      mask TypeOptions Arm_number: Arm_no/Value
      mask TypeOptions Arm_hub_position: Hub_position/Value
      mask TypeOptions eta_dir: eta_dir/Gain
      mask TypeOptions gamma_dir: gamma_dir/Gain
      mask TypeOptions h_prop: h arm/Value
  Cross Product : vrlib/Utilities/Cross Product
  ESC+Motor Dynamcis : XXCopter/ESC+Motor Dynamcis  Inertia_swithc_var=None  J_T=J_T  tau=tau
  F_b->F_A : Product  Multiplication=Matrix(*)
  Ground : Ground
  Gyroscopic Moments : Subsystem  AncestorBlock=XXCopter/Gyroscopic Moments  TreatAsAtomicUnit=on  mask{arm_axis=[0;l_arm;0], Rot_sign=Rot_sign, eta_dir=eta_dir, gamma_dir=gamma_dir, J_T=J_T, J_FA=J_FA}
      mask prompts: arm_axis "Arm axis from Servo origin"; Rot_sign "Rotation sign"; eta_dir "eta direction"; gamma_dir "gamma direction"; J_T "Inertia Motor+Prop"; J_FA "Inertia Foreamr"
      mask TypeOptions arm_axis: arm_axis/Value
      mask TypeOptions Rot_sign: Rotation_sign/Value | Rotation_sign1/Value
      mask TypeOptions eta_dir: eta_dir/Gain | eta_dir1/Gain
      mask TypeOptions gamma_dir: gamma_dir/Gain | gamma_dir1/Gain
      mask TypeOptions J_T: Propeller and motor inertia/Value | Propeller and motor inertia1/Value
      mask TypeOptions J_FA: Forearm Inertia/Value | Forearm Inertia1/Value
  Initial_torque : Memory  X0=Torq_ini
  Permute Dimensions : PermuteDimensions
  Servos Dynamics : XXCopter/Servos Dynamics  omega_n=omega_n  xi=xi  derv_param=c  init_eta=init_eta  init_gamma=0
  Total moments : Sum
  V^A (m/s) : Sum  Inputs=+++
  initial_omega : Memory  X0=Omega_ini
  omega_A : Sum
  omega_b1 : InportShadow  Port=5
  Forces : Outport
  Moments : Outport  Port=2
  Omega_out : Outport  Port=3
  Omega_dot_out : Outport  Port=4
  T_FaFb : Outport  Port=5
  Angles (rad) : Outport  Port=6
  r_p : Outport  Port=7
  wires:
  F_b->F_A/1 -> Aerodynamics Propeller/4(V^A)
  Permute Dimensions/1 -> F_b->F_A/1
  V^A (m/s)/1 -> F_b->F_A/2
  initial_omega/1 -> ESC+Motor Dynamcis/2
  Initial_torque/1 -> ESC+Motor Dynamcis/4
  Aerodynamics Propeller/1(Prop_Torque_out) -> Initial_torque/1
  Total moments/1 -> Moments/1
  Gyroscopic Moments/1(M_gyro @Fb) -> Total moments/2
  Aerodynamics Propeller/3(Moments_prop @Fb) -> Total moments/1
  Ground/1 -> Servos Dynamics/2
  Servos Dynamics/3 -> Gyroscopic Moments/5(Angles_dot _dot(rad/s^2))
  omega_A/1 -> Gyroscopic Moments/2(omega_A  (rad/s))
  omega_b1/1 -> omega_A/2, Gyroscopic Moments/3(omega_b  (rad/s))
  Arms Kinematics/4(omega_Ab (rad/s)) -> omega_A/1
  Servos Dynamics/2 -> Arms Kinematics/2(Angles_dot (rad/s)), Gyroscopic Moments/4(Angles_dot (rad/s))
  Aerodynamics Propeller/2(Forces_prop @Fb) -> Forces/1
  Arms Kinematics/1(r_p (m)) -> r_p/1, Cross Product/2, Aerodynamics Propeller/3(r_p)
  Arms Kinematics/3(T_F_a,Fb) -> Permute Dimensions/1, T_FaFb/1, Aerodynamics Propeller/5(T_FaFb), Gyroscopic Moments/1(T_FAFb)
  Arms Kinematics/2(r_p_dot (m/s)) -> V^A (m/s)/3
  V_b/1 -> V^A (m/s)/1
  Cross Product/1 -> V^A (m/s)/2
  omega_b/1 -> Cross Product/1
  Servos Dynamics/1 -> Angles (rad)/1, Arms Kinematics/1(Angles (rad))
  Comm Angles (rad)/1 -> Servos Dynamics/1
  h_ground/1 -> Aerodynamics Propeller/2(h_ground)
  ESC+Motor Dynamcis/1 -> Aerodynamics Propeller/1(Omega), Omega_out/1, Gyroscopic Moments/6(Omega (rad/s)), initial_omega/1  "Omega"
  ESC+Motor Dynamcis/2 -> Omega_dot_out/1, Gyroscopic Moments/7(Omega_dot (rad/s^2))  "Omega_dot"
  Omega_Initial/1 -> ESC+Motor Dynamcis/3
  Throttle [0-1]/1 -> ESC+Motor Dynamcis/1

== system Validation_Tricopter_Model/3 Copter Complete/Arms Dynamics: Forces and Moments/9 DOF Arms Dynamics: Forces and Moments/9 DOF Arms Dynamics: Forces and Moments/Arm Dynamics2 ==
  note: Motor-Propeller Coupling: Propeller Torque
  Throttle [0-1] : Inport
  Comm Angles (rad) : Inport  Port=2
  Omega_Initial : Inport  Port=3
  h_ground : Inport  Port=4
  omega_b : Inport  Port=5
  V_b : Inport  Port=6
  Aerodynamics Propeller : Subsystem  TreatAsAtomicUnit=on  mask{Rot_sign=Rot_sign}
      mask prompts: Rot_sign "Rotation Sign"
      settings: MinAlgLoopOccurrences=on
      mask TypeOptions Rot_sign: Rotation_sign/Value
  Arms Kinematics : Subsystem  AncestorBlock=XXCopter/Arms Kinematics  TreatAsAtomicUnit=on  mask{Arm_number=arm_num, Arm_hub_position=arm_hub_pos, eta_dir=eta_dir, gamma_dir=gamma_dir, h_prop=h}
      mask prompts: Arm_number "Arm number (1,2 or 3)"; Arm_hub_position "Arm Hub position"; eta_dir "eta direcction"; gamma_dir "gamma diretion"; h_prop "h of propeller hub"
      mask help:
      | If Arm number 1 (Forward one)
      | eta_dir=[1,0,0]
      | gamma_dir=[0,1,0]
      |
      | If Arm number 2 or 3 (rear ones)
      | eta_dir=[0,1,0]
      | gamma_dir=[1,0,0]
      mask TypeOptions Arm_number: Arm_no/Value
      mask TypeOptions Arm_hub_position: Hub_position/Value
      mask TypeOptions eta_dir: eta_dir/Gain
      mask TypeOptions gamma_dir: gamma_dir/Gain
      mask TypeOptions h_prop: h arm/Value
  Cross Product : vrlib/Utilities/Cross Product
  ESC+Motor Dynamcis : XXCopter/ESC+Motor Dynamcis  Inertia_swithc_var=None  J_T=J_T  tau=tau
  F_b->F_A : Product  Multiplication=Matrix(*)
  Ground : Ground
  Gyroscopic Moments : Subsystem  AncestorBlock=XXCopter/Gyroscopic Moments  TreatAsAtomicUnit=on  mask{arm_axis=[0;-l_arm;0], Rot_sign=Rot_sign, eta_dir=eta_dir, gamma_dir=gamma_dir, J_T=J_T, J_FA=J_FA}
      mask prompts: arm_axis "Arm axis from Servo origin"; Rot_sign "Rotation sign"; eta_dir "eta direction"; gamma_dir "gamma direction"; J_T "Inertia Motor+Prop"; J_FA "Inertia Foreamr"
      mask TypeOptions arm_axis: arm_axis/Value
      mask TypeOptions Rot_sign: Rotation_sign/Value | Rotation_sign1/Value
      mask TypeOptions eta_dir: eta_dir/Gain | eta_dir1/Gain
      mask TypeOptions gamma_dir: gamma_dir/Gain | gamma_dir1/Gain
      mask TypeOptions J_T: Propeller and motor inertia/Value | Propeller and motor inertia1/Value
      mask TypeOptions J_FA: Forearm Inertia/Value | Forearm Inertia1/Value
  Initial_torque : Memory  X0=Torq_ini
  Permute Dimensions : PermuteDimensions
  Servos Dynamics : XXCopter/Servos Dynamics  omega_n=omega_n  xi=xi  derv_param=c  init_eta=init_eta  init_gamma=0
  Total moments : Sum
  V^A (m/s) : Sum  Inputs=+++
  initial_omega : Memory  X0=Omega_ini
  omega_A : Sum
  omega_b1 : InportShadow  Port=5
  Forces : Outport
  Moments : Outport  Port=2
  Omega_out : Outport  Port=3
  Omega_dot_out : Outport  Port=4
  T_FaFb : Outport  Port=5
  Angles (rad) : Outport  Port=6
  r_p : Outport  Port=7
  wires:
  F_b->F_A/1 -> Aerodynamics Propeller/4(V^A)
  Permute Dimensions/1 -> F_b->F_A/1
  V^A (m/s)/1 -> F_b->F_A/2
  initial_omega/1 -> ESC+Motor Dynamcis/2
  Initial_torque/1 -> ESC+Motor Dynamcis/4
  Aerodynamics Propeller/1(Prop_Torque_out) -> Initial_torque/1
  Total moments/1 -> Moments/1
  Gyroscopic Moments/1(M_gyro @Fb) -> Total moments/2
  Aerodynamics Propeller/3(Moments_prop @Fb) -> Total moments/1
  Ground/1 -> Servos Dynamics/2
  Servos Dynamics/3 -> Gyroscopic Moments/5(Angles_dot _dot(rad/s^2))
  omega_A/1 -> Gyroscopic Moments/2(omega_A  (rad/s))
  omega_b1/1 -> omega_A/2, Gyroscopic Moments/3(omega_b  (rad/s))
  Arms Kinematics/4(omega_Ab (rad/s)) -> omega_A/1
  Servos Dynamics/2 -> Arms Kinematics/2(Angles_dot (rad/s)), Gyroscopic Moments/4(Angles_dot (rad/s))
  Aerodynamics Propeller/2(Forces_prop @Fb) -> Forces/1
  Arms Kinematics/1(r_p (m)) -> r_p/1, Cross Product/2, Aerodynamics Propeller/3(r_p)
  Arms Kinematics/3(T_F_a,Fb) -> Permute Dimensions/1, T_FaFb/1, Aerodynamics Propeller/5(T_FaFb), Gyroscopic Moments/1(T_FAFb)
  Arms Kinematics/2(r_p_dot (m/s)) -> V^A (m/s)/3
  V_b/1 -> V^A (m/s)/1
  Cross Product/1 -> V^A (m/s)/2
  omega_b/1 -> Cross Product/1
  Servos Dynamics/1 -> Angles (rad)/1, Arms Kinematics/1(Angles (rad))
  Comm Angles (rad)/1 -> Servos Dynamics/1
  h_ground/1 -> Aerodynamics Propeller/2(h_ground)
  ESC+Motor Dynamcis/1 -> Aerodynamics Propeller/1(Omega), Omega_out/1, Gyroscopic Moments/6(Omega (rad/s)), initial_omega/1  "Omega"
  ESC+Motor Dynamcis/2 -> Omega_dot_out/1, Gyroscopic Moments/7(Omega_dot (rad/s^2))  "Omega_dot"
  Omega_Initial/1 -> ESC+Motor Dynamcis/3
  Throttle [0-1]/1 -> ESC+Motor Dynamcis/1

== system Validation_Tricopter_Model/Controller/NDI+CA Controller/ 9DOF NDI+CA Controller - No massic update/Control Allocation 9DOF/Control Allocation 9DOF ==
  note: Enabler override saturations and override
      | them with zero to avoid actuators being
      | locked by control allocation algorithm
  note: Weights used to normalize different
      | inputs between controllers.
      | Throttle - 0 to 1
      | Servo - 0 to 2*pi
  note: Position and rate limits for
      | tricopter actuators
  Pseudocontrol input : Inport
  Effectiveness control matrix : Inport  Port=2
  "Control allocator Completed " : qcatlib/Control allocator Completed   alg=WLS  CA_type=QP  iter_max=4  gamma=1e6  k_B=6  m_B=9  T=0.01  tol=0
  Control desired (0 to minimize control effort) : Constant  Value=zeros(1,9)
  Control desired (Timmed 9DOF) : Constant  Value=[0.6049, -0.7465,-0.07355,0.6044,-0.7422,0.4171,0.6044,0.5941,0.417]
  Control positions deviation Weight W1 : Constant  Value=diag(1./[1,2*pi,2*pi,1,2*pi,2*pi,1,2*pi,2*pi] )
  Control rate deviation Weight W2 : Constant  Value=diag(1./[1,2*pi,2*pi,1,2*pi,2*pi,1,2*pi,2*pi] )
  Enalbe/Disable : Constant
  Error Weight Wv2 : Constant  Value=blkdiag(1,1,1, 1/(2*pi), 1/(2*pi), 1/(2*pi))
  Position limits 9DOF : Constant  Value=[ [0,-deg2rad(165),-deg2rad(90),0,-deg2rad(165),-deg2rad(15),0,-deg2rad(165),-deg2rad(90)]', [1,deg2rad(165),deg2rad(15),1,deg2rad(165),deg2rad(90),1,deg2rad(165),deg2rad(15)]']
  Rates limits 9DOF : Constant  Value=[ [-17,-1,-1,-17,-1,-1,-17,-1,-1]', [17,1,1,17,1,1,17,1,1]']*2
  Reshape1 : Reshape  OutputDimensionality=Customize  OutputDimensions=[6,9]
  Reshape2 : Reshape  OutputDimensions=[6,1]
  Terminator : Terminator
  Terminator1 : Terminator
  Unit Delay : UnitDelay  SampleTime=-1
  manual Initial saturations : Constant  Value=zeros(9,1)
  Control output : Outport  PortDimensions=9
  wires:
  "Control allocator Completed "/2 -> Terminator/1
  "Control allocator Completed "/3 -> Terminator1/1
  Effectiveness control matrix/1 -> Reshape1/1
  Reshape1/1 -> "Control allocator Completed "/4
  Position limits 9DOF/1 -> "Control allocator Completed "/5
  Rates limits 9DOF/1 -> "Control allocator Completed "/6
  Error Weight Wv2/1 -> "Control allocator Completed "/7
  Control positions deviation Weight W1/1 -> "Control allocator Completed "/8
  Control rate deviation Weight W2/1 -> "Control allocator Completed "/9
  manual Initial saturations/1 -> "Control allocator Completed "/10
  Enalbe/Disable/1 -> "Control allocator Completed "/11
  Reshape2/1 -> Control output/1
  "Control allocator Completed "/1 -> Reshape2/1, Unit Delay/1
  Unit Delay/1 -> "Control allocator Completed "/2
  Pseudocontrol input/1 -> "Control allocator Completed "/1
  Control desired (Timmed 9DOF)/1 -> "Control allocator Completed "/3

== system Validation_Tricopter_Model/Controller/NDI+CA Controller/ 9DOF NDI+CA Controller - No massic update/Control Allocation 9DOF/Pseudoinverse 9DOF ==
  Pseudocontrol input : Inport
  Effectiveness control matrix : Inport  Port=2
  Product1 : Product  Multiplication=Matrix(*)
  Pseudoinverse : dspinverses/Pseudoinverse  wanterr=off
  Reshape1 : Reshape  OutputDimensions=[6,1]
  Control output : Outport  PortDimensions=9
  wires:
  Product1/1 -> Reshape1/1
  Pseudoinverse/1 -> Product1/1
  Effectiveness control matrix/1 -> Pseudoinverse/1
  Pseudocontrol input/1 -> Product1/2
  Reshape1/1 -> Control output/1
